simulink model "sensorExpoler_Encoderslx"  (R2026a)
settings: Solver=FixedStepDiscrete  StopTime=32  FixedStep=0.0001
undefined symbols (not defined in the file): Blocking, Non
libraries: simulink x3, amg_usbconverter_n_connect_lib x2
settings Model: Creator=pboon  LastModifiedBy=matthurindo

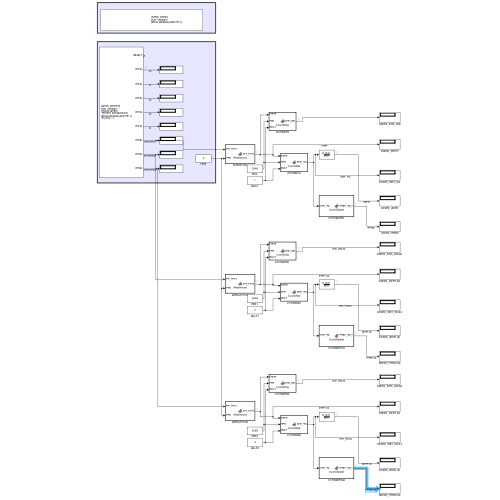
[thumbnail: Simulink's stored preview of the top-level diagram]
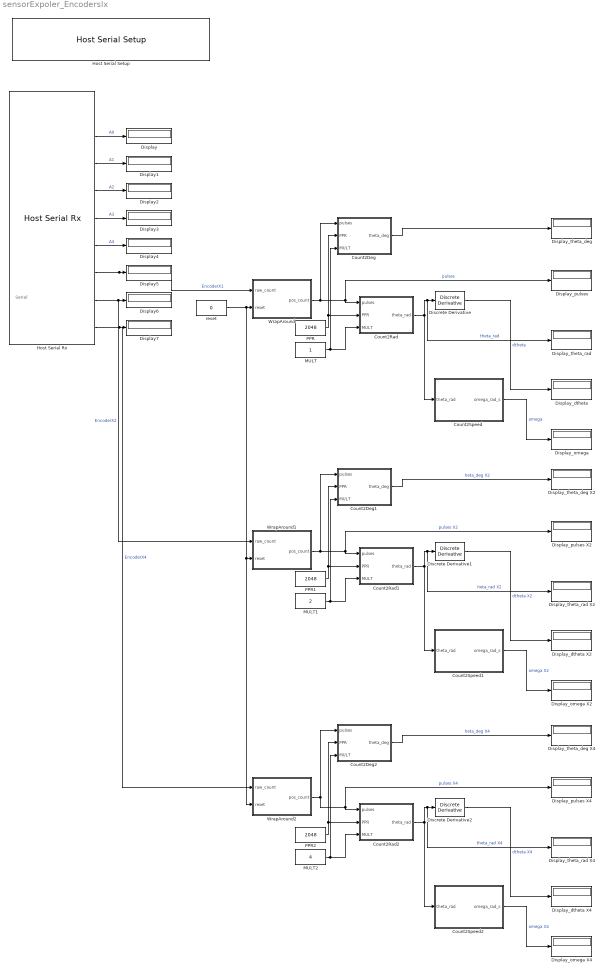
== system sensorExpoler_Encoderslx ==
  note: Serial
  Count2Deg : MATLAB Function  TreatAsAtomicUnit=on
  Count2Deg1 : MATLAB Function  TreatAsAtomicUnit=on
  Count2Deg2 : MATLAB Function  TreatAsAtomicUnit=on
  Count2Rad : MATLAB Function  TreatAsAtomicUnit=on
  Count2Rad1 : MATLAB Function  TreatAsAtomicUnit=on
  Count2Rad2 : MATLAB Function  TreatAsAtomicUnit=on
  Count2Speed : MATLAB Function  TreatAsAtomicUnit=on
  Count2Speed1 : MATLAB Function  TreatAsAtomicUnit=on
  Count2Speed2 : MATLAB Function  TreatAsAtomicUnit=on
  Discrete Derivative : simulink/Discrete/Discrete Derivative  gainval=1.0  ICPrevScaledInput=0.0  OutMin=[]  OutMax=[]  OutDataType=fixdt(1, 16)  OutScaling=2^-10  DoSatur=off
  Discrete Derivative1 : simulink/Discrete/Discrete Derivative  gainval=1.0  ICPrevScaledInput=0.0  OutMin=[]  OutMax=[]  OutDataType=fixdt(1, 16)  OutScaling=2^-10  DoSatur=off
  Discrete Derivative2 : simulink/Discrete/Discrete Derivative  gainval=1.0  ICPrevScaledInput=0.0  OutMin=[]  OutMax=[]  OutDataType=fixdt(1, 16)  OutScaling=2^-10  DoSatur=off
  Display{,1..7} (8 alike) : Display
  Display_dtheta : Display
  Display_dtheta X2 : Display
  Display_dtheta X4 : Display
  Display_omega : Display
  Display_omega X2 : Display
  Display_omega X4 : Display
  Display_pulses : Display
  Display_pulses X2 : Display
  Display_pulses X4 : Display
  Display_theta_deg : Display
  Display_theta_deg X2 : Display
  Display_theta_deg X4 : Display
  Display_theta_rad : Display
  Display_theta_rad X2 : Display
  Display_theta_rad X4 : Display
  Host Serial Rx : amg_usbconverter_n_connect_lib/Host Serial Rx  conf=rx  port=<auto>  baudrate=2000000  databits=8  parity=None  stopbit=1  flowcontrol=None  transfer=Non-Blocking  timeout=5  packetmode=Binary  enableinitialvalues=off  initialvalues=[]  binheader='25'  binterminator='4E 4E'  porttype_double=0  porttype_single=0  porttype_int8=0  porttype_uint8=0  porttype_int16=0  porttype_uint16=5  porttype_int32=0  porttype_uint32=3  asciiformat='%d,%f'  rx_asciiterminator="CRLF (0x0D 0x0A - \"\\r\\n\")"  tx_asciiterminator="CRLF (0x0D 0x0A - \"\\r\\n\")"  sampletime=0.001  enablecustomportlabel=off  cinputportlabel=0  coutputportlabel=A  portpinstr=0  blockid=HostSerialRx  inputporttype=[]  inputportwidth=[]  inputportlabel={}  outputporttype=[3 5 5 5 5 5 7 7 7]  outputportwidth=[1 1 1 1 1 1 1 1 1]  outputportlabel={'READY','uint16','uint16','uint16','uint16','uint16','uint32','uint32','uint32'}  compat=0  optionstring=[]  autoport='<empty>'
  Host Serial Setup : amg_usbconverter_n_connect_lib/Host Serial Setup  conf=setup  port=<auto>  baudrate=2000000  databits=8  parity=None  stopbit=1  flowcontrol=None  transfer=Blocking  timeout=2  packetmode=Binary  initialvalues=[]  binheader='7E 7E'  binterminator='03 03'  porttype_double=0  porttype_single=1  porttype_int8=0  porttype_uint8=0  porttype_int16=0  porttype_uint16=0  porttype_int32=0  porttype_uint32=2  asciiformat='%d %u %x'  rx_asciiterminator="CRLF (0x0D 0x0A - \"\\r\\n\")"  tx_asciiterminator="CRLF (0x0D 0x0A - \"\\r\\n\")"  sampletime=-1  enablecustomportlabel=off  cinputportlabel=0  coutputportlabel=A  portpinstr=0  blockid=HostSerialSetup  inputporttype=[]  inputportwidth=[]  inputportlabel={}  outputporttype=[]  outputportwidth=[]  outputportlabel={}  compat=0  optionstring=[]  autoport='<empty>'
  MULT : Constant
  MULT1 : Constant  Value=2
  MULT2 : Constant  Value=4
  PPR : Constant  Value=2048
  PPR1 : Constant  Value=2048
  PPR2 : Constant  Value=2048
  WrapAround : MATLAB Function  TreatAsAtomicUnit=on
  WrapAround1 : MATLAB Function  TreatAsAtomicUnit=on
  WrapAround2 : MATLAB Function  TreatAsAtomicUnit=on
  reset : Constant  Value=0
  wires:
  Host Serial Rx/2 -> Display/1  "A0"
  Host Serial Rx/3 -> Display1/1  "A1"
  Host Serial Rx/4 -> Display2/1  "A2"
  Host Serial Rx/5 -> Display3/1  "A3"
  Host Serial Rx/6 -> Display4/1  "A4"
  Host Serial Rx/7 -> WrapAround/1(raw_count), Display5/1  "EncoderX1"
  Host Serial Rx/8 -> WrapAround1/1(raw_count), Display6/1  "EncoderX2"
  Host Serial Rx/9 -> WrapAround2/1(raw_count), Display7/1  "EncoderX4"
  reset/1 -> WrapAround1/2(reset), WrapAround2/2(reset), WrapAround/2(reset)
  PPR/1 -> Count2Rad/2(PPR), Count2Deg/2(PPR)
  MULT/1 -> Count2Rad/3(MULT), Count2Deg/3(MULT)
  WrapAround/1(pos_count) -> Count2Rad/1(pulses), Display_pulses/1, Count2Deg/1(pulses)  "pulses"
  Count2Rad/1(theta_rad) -> Discrete Derivative/1, Display_theta_rad/1, Count2Speed/1(theta_rad)  "theta_rad"
  Count2Deg/1(theta_deg) -> Display_theta_deg/1
  Discrete Derivative/1 -> Display_dtheta/1  "dtheta"
  Count2Speed/1(omega_rad_s) -> Display_omega/1  "omega"
  Discrete Derivative1/1 -> Display_dtheta X2/1  "dtheta X2"
  WrapAround1/1(pos_count) -> Count2Rad1/1(pulses), Display_pulses X2/1, Count2Deg1/1(pulses)  "pulses X2"
  MULT1/1 -> Count2Rad1/3(MULT), Count2Deg1/3(MULT)
  Count2Rad1/1(theta_rad) -> Discrete Derivative1/1, Display_theta_rad X2/1, Count2Speed1/1(theta_rad)  "heta_rad X2"
  Count2Deg1/1(theta_deg) -> Display_theta_deg X2/1  "heta_deg X2"
  Count2Speed1/1(omega_rad_s) -> Display_omega X2/1  "omega X2"
  PPR1/1 -> Count2Rad1/2(PPR), Count2Deg1/2(PPR)
  Discrete Derivative2/1 -> Display_dtheta X4/1  "dtheta X4"
  WrapAround2/1(pos_count) -> Count2Rad2/1(pulses), Display_pulses X4/1, Count2Deg2/1(pulses)  "pulses X4"
  MULT2/1 -> Count2Rad2/3(MULT), Count2Deg2/3(MULT)
  Count2Rad2/1(theta_rad) -> Discrete Derivative2/1, Display_theta_rad X4/1, Count2Speed2/1(theta_rad)  "theta_rad X4"
  Count2Deg2/1(theta_deg) -> Display_theta_deg X4/1  "heta_deg X4"
  Count2Speed2/1(omega_rad_s) -> Display_omega X4/1  "omega X4"
  PPR2/1 -> Count2Rad2/2(PPR), Count2Deg2/2(PPR)

== matlab function sensorExpoler_Encoderslx/Count2Rad ==
  data: pulses input; theta_rad output; PPR input; MULT input
function theta_rad = Count2Rad(pulses, PPR, MULT)
theta_rad = (pulses / (PPR * MULT)) * 2*pi;

== matlab function sensorExpoler_Encoderslx/WrapAround2 ==
  data: raw_count input; pos_count output; reset input
function pos_count = WrapAround(raw_count, reset)
persistent prev acc nBlank
MAX_COUNT = 65536;
MAXC = double(MAX_COUNT);
raw = mod(double(raw_count), MAXC);
if isempty(prev)
    prev = raw; acc = 0; nBlank = 0;
end
BLANK_SAMPLES = 150;
if reset ~= 0
    acc = 0; prev = raw; nBlank = 0;
    pos_count = acc; return
end
if nBlank < BLANK_SAMPLES
    nBlank = nBlank + 1; prev = raw;
    pos_count = acc; return
end
delta = raw - prev;
if delta > MAXC/2
    delta = delta - MAXC;
elseif delta < -MAXC/2
    delta = delta + MAXC;
end
acc = acc + delta;
prev = raw;
pos_count = acc;

== matlab function sensorExpoler_Encoderslx/Count2Deg ==
  data: pulses input; theta_deg output; PPR input; MULT input
function theta_deg = Count2Deg(pulses, PPR, MULT)
theta_deg = (pulses / (PPR * MULT)) * 360;

== matlab function sensorExpoler_Encoderslx/WrapAround ==
  data: raw_count input; pos_count output; reset input
function pos_count = WrapAround(raw_count, reset)
persistent prev acc nBlank
MAX_COUNT = 65536;
MAXC = double(MAX_COUNT);
raw = mod(double(raw_count), MAXC);
if isempty(prev)
    prev = raw; acc = 0; nBlank = 0;
end
BLANK_SAMPLES = 150;
if reset ~= 0
    acc = 0; prev = raw; nBlank = 0;
    pos_count = acc; return
end
if nBlank < BLANK_SAMPLES
    nBlank = nBlank + 1; prev = raw;
    pos_count = acc; return
end
delta = raw - prev;
if delta > MAXC/2
    delta = delta - MAXC;
elseif delta < -MAXC/2
    delta = delta + MAXC;
end
acc = acc + delta;
prev = raw;
pos_count = acc;

== matlab function sensorExpoler_Encoderslx/Count2Speed ==
  data: theta_rad input; omega_rad_s output
function omega_rad_s = Count2Speed(theta_rad)
%#codegen
% Count2Speed -- angular velocity [rad/s], backward difference + first-order
% exponential smoothing.  Paste into a MATLAB Function block named
% "Count2Speed".
%
% Ports   theta_rad : from Count2Rad
%         Ts        : sample time [s] -- 0.001 in this lab (Constant block)
%         alpha     : smoothing factor, 0 < alpha <= 1 (Constant block)
%                       1.0  = raw 1 ms difference (very spiky, see below)
%                       0.05 = ~20 ms time constant at Ts = 1 ms  <- good
%                              starting point for the report figures
%         -> omega_rad_s  (0 until the second sample)
%
% Why smoothing is not optional here:
%   One count = 2*pi/countsPerRev rad.  At Ts = 1 ms that is a 3.07 rad/s
%   quantization step for AMT X1 (0.77 for X4, 262 for Bourns X1).  The
%   recorded AMT runs also update in bursts: after the first 0.5 s the
%   median |raw step| is 0-1 counts but single-sample steps reach 99-232
%   counts, so an unsmoothed 1 ms derivative is dominated by spikes.
%   For a single steady-state number, use the average over the moving part
%   of the run instead:  omega_avg = (theta_end - theta_start)/(t_end - t_start).
%
% If you want a different filter (moving average, Discrete FIR Filter,
% Discrete Derivative + Low Pass Filter), you can skip this block entirely.
persistent prev w
Ts = 0.001;
alpha = 1;
if isempty(prev)
    prev = theta_rad; w = 0;
end
if nargin < 3 || isempty(alpha)
    alpha = 1;
end
alpha = min(max(alpha, 0), 1);      % clamp to [0,1]
raw_w = (theta_rad - prev) / Ts;
w     = w + alpha * (raw_w - w);
prev  = theta_rad;
omega_rad_s = w;

== matlab function sensorExpoler_Encoderslx/Count2Deg1 ==
  data: pulses input; theta_deg output; PPR input; MULT input
function theta_deg = Count2Deg(pulses, PPR, MULT)
theta_deg = (pulses / (PPR * MULT)) * 360;

== matlab function sensorExpoler_Encoderslx/Count2Rad1 ==
  data: pulses input; theta_rad output; PPR input; MULT input
function theta_rad = Count2Rad(pulses, PPR, MULT)
theta_rad = (pulses / (PPR * MULT)) * 2*pi;

== matlab function sensorExpoler_Encoderslx/Count2Speed1 ==
  data: theta_rad input; omega_rad_s output
function omega_rad_s = Count2Speed(theta_rad)
%#codegen
% Count2Speed -- angular velocity [rad/s], backward difference + first-order
% exponential smoothing.  Paste into a MATLAB Function block named
% "Count2Speed".
%
% Ports   theta_rad : from Count2Rad
%         Ts        : sample time [s] -- 0.001 in this lab (Constant block)
%         alpha     : smoothing factor, 0 < alpha <= 1 (Constant block)
%                       1.0  = raw 1 ms difference (very spiky, see below)
%                       0.05 = ~20 ms time constant at Ts = 1 ms  <- good
%                              starting point for the report figures
%         -> omega_rad_s  (0 until the second sample)
%
% Why smoothing is not optional here:
%   One count = 2*pi/countsPerRev rad.  At Ts = 1 ms that is a 3.07 rad/s
%   quantization step for AMT X1 (0.77 for X4, 262 for Bourns X1).  The
%   recorded AMT runs also update in bursts: after the first 0.5 s the
%   median |raw step| is 0-1 counts but single-sample steps reach 99-232
%   counts, so an unsmoothed 1 ms derivative is dominated by spikes.
%   For a single steady-state number, use the average over the moving part
%   of the run instead:  omega_avg = (theta_end - theta_start)/(t_end - t_start).
%
% If you want a different filter (moving average, Discrete FIR Filter,
% Discrete Derivative + Low Pass Filter), you can skip this block entirely.
persistent prev w
Ts = 0.001;
alpha = 1;
if isempty(prev)
    prev = theta_rad; w = 0;
end
if nargin < 3 || isempty(alpha)
    alpha = 1;
end
alpha = min(max(alpha, 0), 1);      % clamp to [0,1]
raw_w = (theta_rad - prev) / Ts;
w     = w + alpha * (raw_w - w);
prev  = theta_rad;
omega_rad_s = w;

== matlab function sensorExpoler_Encoderslx/WrapAround1 ==
  data: raw_count input; pos_count output; reset input
function pos_count = WrapAround(raw_count, reset)
persistent prev acc nBlank
MAX_COUNT = 65536;
MAXC = double(MAX_COUNT);
raw = mod(double(raw_count), MAXC);
if isempty(prev)
    prev = raw; acc = 0; nBlank = 0;
end
BLANK_SAMPLES = 150;
if reset ~= 0
    acc = 0; prev = raw; nBlank = 0;
    pos_count = acc; return
end
if nBlank < BLANK_SAMPLES
    nBlank = nBlank + 1; prev = raw;
    pos_count = acc; return
end
delta = raw - prev;
if delta > MAXC/2
    delta = delta - MAXC;
elseif delta < -MAXC/2
    delta = delta + MAXC;
end
acc = acc + delta;
prev = raw;
pos_count = acc;

== matlab function sensorExpoler_Encoderslx/Count2Deg2 ==
  data: pulses input; theta_deg output; PPR input; MULT input
function theta_deg = Count2Deg(pulses, PPR, MULT)
theta_deg = (pulses / (PPR * MULT)) * 360;

== matlab function sensorExpoler_Encoderslx/Count2Rad2 ==
  data: pulses input; theta_rad output; PPR input; MULT input
function theta_rad = Count2Rad(pulses, PPR, MULT)
theta_rad = (pulses / (PPR * MULT)) * 2*pi;

== matlab function sensorExpoler_Encoderslx/Count2Speed2 ==
  data: theta_rad input; omega_rad_s output
function omega_rad_s = Count2Speed(theta_rad)
%#codegen
% Count2Speed -- angular velocity [rad/s], backward difference + first-order
% exponential smoothing.  Paste into a MATLAB Function block named
% "Count2Speed".
%
% Ports   theta_rad : from Count2Rad
%         Ts        : sample time [s] -- 0.001 in this lab (Constant block)
%         alpha     : smoothing factor, 0 < alpha <= 1 (Constant block)
%                       1.0  = raw 1 ms difference (very spiky, see below)
%                       0.05 = ~20 ms time constant at Ts = 1 ms  <- good
%                              starting point for the report figures
%         -> omega_rad_s  (0 until the second sample)
%
% Why smoothing is not optional here:
%   One count = 2*pi/countsPerRev rad.  At Ts = 1 ms that is a 3.07 rad/s
%   quantization step for AMT X1 (0.77 for X4, 262 for Bourns X1).  The
%   recorded AMT runs also update in bursts: after the first 0.5 s the
%   median |raw step| is 0-1 counts but single-sample steps reach 99-232
%   counts, so an unsmoothed 1 ms derivative is dominated by spikes.
%   For a single steady-state number, use the average over the moving part
%   of the run instead:  omega_avg = (theta_end - theta_start)/(t_end - t_start).
%
% If you want a different filter (moving average, Discrete FIR Filter,
% Discrete Derivative + Low Pass Filter), you can skip this block entirely.
persistent prev w
Ts = 0.001;
alpha = 1;
if isempty(prev)
    prev = theta_rad; w = 0;
end
if nargin < 3 || isempty(alpha)
    alpha = 1;
end
alpha = min(max(alpha, 0), 1);      % clamp to [0,1]
raw_w = (theta_rad - prev) / Ts;
w     = w + alpha * (raw_w - w);
prev  = theta_rad;
omega_rad_s = w;
